simulink model "GalvoModel_v44_simply"  (R2013a)
settings: Solver=ode45  StartTime=0.0  StopTime=10.0  MaxStep=1e-4  RelTol=1e-3
InitFcn:
  | param=evalin('base','param;');
  | 
  | JR=str2num(param.JR);
  | KMT=str2num(param.KMT);
  | Rc=str2num(param.Rc);
  | Lc=str2num(param.Lc);
  | KFR=str2num(param.KFR);
  | KTB=str2num(param.KTB);
  | KBM=str2num(param.KBM);
  | Rsh=str2num(param.Rsh);
StartFcn:
  | sprintf('Info (%s):\nKTB = %.1e\nKBM = %.1e\n', gcs, KTB, KBM)
model workspace (MATLAB code in the model file):
  | %param=evalin('base','loadGalvoParam(4);');
  | param=evalin('base','param;');
  | 
  | JR=str2num(param.JR);
  | KMT=str2num(param.KMT);
  | Rc=str2num(param.Rc);
  | Lc=str2num(param.Lc);
  | KFR=str2num(param.KFR);
  | KTB=str2num(param.KTB);
  | KBM=str2num(param.KBM);
  | Rsh=str2num(param.Rsh);
undefined symbols (not defined in the file): FS
settings Model: BufferReuse=off  Creator=mainster  LastModifiedBy=mainster
settings DataIOCC: SaveOutput=off  SaveTime=off
settings OptimizationCC: InlineParams=on  BufferReuse=off
settings DebuggingCC: InitInArrayFormatMsg=none
settings ModelReferenceCC: ModelReferenceMinAlgLoopOccurrences=on

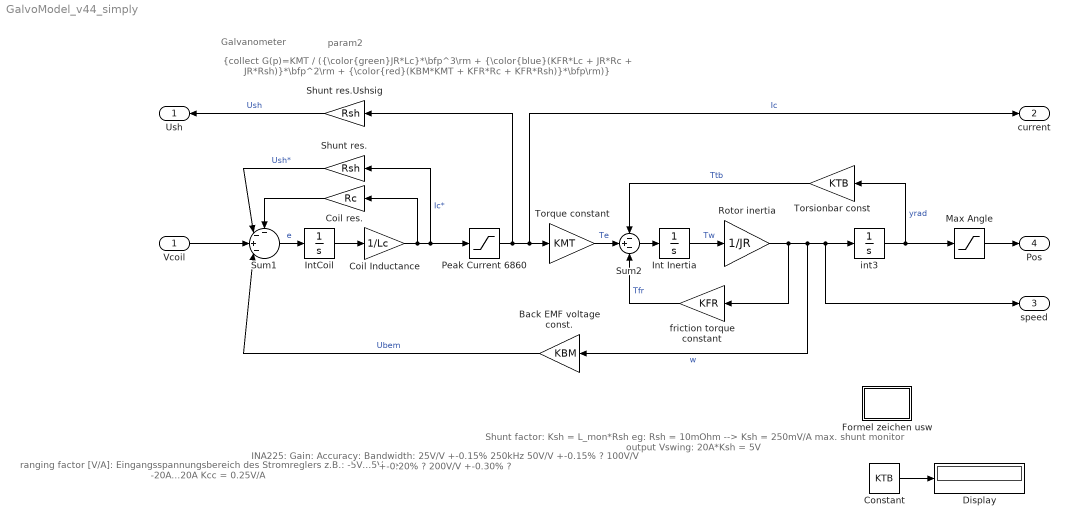
== system GalvoModel_v44_simply ==
  note: {collect G(p)=KMT / ({\color{green}JR*Lc}*\bfp^3\rm + {\color{blue}(KFR*Lc + JR*Rc + JR*Rsh)}*\bfp^2\rm + {\color{red}(KBM*KMT + KFR*Rc + KFR*Rsh)}*\bfp\rm)}
  note: param2
  note: Galvanometer
  note: ranging factor [V/A]:
      | Eingangsspannungsbereich des
      | Stromreglers z.B.:
      | -5V...5V --> -20A...20A
      | Kcc = 0.25V/A
  note: Shunt factor:
      | Ksh = L_mon*Rsh
      |
      | eg: Rsh = 10mOhm
      |
      | --> Ksh = 250mV/A
      | max. shunt monitor
      | output Vswing:
      | 20A*Ksh = 5V
  note: INA225:
      | Gain:		Accuracy:		Bandwidth:
      | 25V/V		+-0.15%		250kHz
      | 50V/V		+-0.15%		?
      | 100V/V	+-0.20%		?
      | 200V/V	+-0.30%		?
  Vcoil : Inport
  Back EMF voltage const. : Gain  Gain=KBM  SampleTime=FS
  Coil Inductance : Gain  Gain=1/Lc  SampleTime=FS
  Coil res. : Gain  Gain=Rc  SampleTime=FS
  Constant : Constant  Value=KTB  SampleTime=FS
  Display : Display
  Formel zeichen usw : Subsystem
  Int Inertia : Integrator
  IntCoil : Integrator
  Max Angle : Saturate  UpperLimit=20*pi/180  LowerLimit=-20*pi/180  SampleTime=FS
      settings: AttributesFormatString=Max=%<UpperLimit>\nMin=%<LowerLimit>
  Peak Current 6860 : Saturate  UpperLimit=30  LowerLimit=-30  SampleTime=FS
      settings: AttributesFormatString=+-%<UpperLimit>A
  Rotor inertia : Gain  Gain=1/JR  SampleTime=FS
  Shunt res. : Gain  Gain=Rsh  SampleTime=FS
  Shunt res.Ushsig : Gain  Gain=Rsh  SampleTime=FS
  Sum1 : Sum  Inputs=--+-|  SampleTime=FS
  Sum2 : Sum  Inputs=-+-  SampleTime=FS
  Torque constant : Gain  Gain=KMT  SampleTime=FS
  Torsionbar const : Gain  Gain=KTB  SampleTime=FS
  friction torque constant : Gain  Gain=KFR  SampleTime=FS
  int3 : Integrator
  Ush : Outport
  current : Outport  Port=2
  speed : Outport  Port=3
  Pos : Outport  Port=4
  wires:
  Shunt res./1 -> Sum1/2  "Ush*"
  Coil res./1 -> Sum1/1
  Vcoil/1 -> Sum1/3
  Back EMF voltage const./1 -> Sum1/4  "Ubem"
  int3/1 -> Max Angle/1, Torsionbar const/1  "yrad"
  Torque constant/1 -> Sum2/2  "Te"
  Coil Inductance/1 -> Coil res./1, Shunt res./1, Peak Current 6860/1  "Ic*"
  Torsionbar const/1 -> Sum2/1  "Ttb"
  IntCoil/1 -> Coil Inductance/1
  Sum1/1 -> IntCoil/1  "e"
  Int Inertia/1 -> Rotor inertia/1  "Tw"
  Sum2/1 -> Int Inertia/1
  Rotor inertia/1 -> friction torque constant/1, speed/1, int3/1, Back EMF voltage const./1  "w"
  friction torque constant/1 -> Sum2/3  "Tfr"
  Constant/1 -> Display/1
  Max Angle/1 -> Pos/1
  Peak Current 6860/1 -> Shunt res.Ushsig/1, current/1, Torque constant/1  "Ic"
  Shunt res.Ushsig/1 -> Ush/1  "Ush"

== system GalvoModel_v44_simply/Formel zeichen usw ==
  note: Te: 		electrical torque, gen. by coils		[Nm]
      |  Ic: 			coil current							[A]
      |  Tfr:		rotor dynamic friction torque 		[Nm]
      |  Trb:		torsion bar torque					[Nm]
      |  Tw:		angular momentum				[Nm*s]
      |  w:			angular velocity 					[rad/s]
      |  yrad:		angular position 					[rad]
      |  ydeg:		angular position 					[°]
      |  Ucci:		current controller input				[V]
      |  Ucco:		current controller output			[V]
      |  Ush:		shunt voltage						[V]
  note: balance of force: 	Te=Ttb+Tfr
      | 					Te - (Ttb+Tfr)=0  ->  no movement
      |
      |  integrate( 1 Nm )dt = 1 Nm*s
      |  (Nm*s)(kg*m²)⁻¹ = (N*s/kg)*m⁻¹ = m/(s*m) = rad
  note: L_{c  }	coil inductance 							[H]
      |  R_{c  }	coil resistance							[\Omega]
      |  R_{SH }	current shunt resistance				[\Omega]
      |  J_{R  }	rotor inertia 							[kg*m²]
      |  \color{red}K_{TB }	torsion bar torque const. 			[Nm/rad]
      |  \color{black}K_{BM }	back EMF const.							[V*s/rad]
      |  K_{FR }	rotor dyn. friction torque const.	[Nm*s/rad]
      |  K_{MT }	el. magnetic torque const.			[Nm/A]
